simulink model "test1"  (Simulink 7.8)
settings: Solver=ode45  StartTime=0.0  StopTime=10.0  RelTol=1e-3
settings Model: Creator=Magnifico  LastModifiedBy=Magnifico

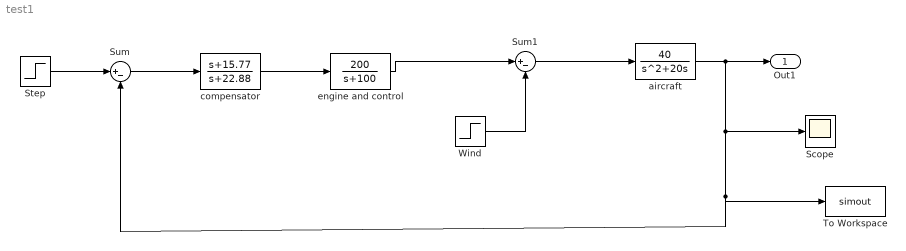
== system test1 ==
  Scope : Scope
  Step : Step  SampleTime=0
  Sum : Sum  Inputs=|+-
  Sum1 : Sum  Inputs=|+-
  To Workspace : ToWorkspace  VariableName=simout  SampleTime=-1  SaveFormat=Structure
  Wind : Step  SampleTime=0
  aircraft : TransferFcn  Numerator=[40]  Denominator=[1 20 0]
  compensator : TransferFcn  Numerator=[1 15.77]  Denominator=[1 22.88]
  engine and control : TransferFcn  Numerator=[200]  Denominator=[1 100]
  Out1 : Outport
  wires:
  Sum/1 -> compensator/1
  Step/1 -> Sum/1
  Sum1/1 -> aircraft/1
  engine and control/1 -> Sum1/1
  compensator/1 -> engine and control/1
  aircraft/1 -> Out1/1, Scope/1, Sum/2, To Workspace/1
  Wind/1 -> Sum1/2
